simulink model "untitled"  (R2019a)
settings: Solver=VariableStepAuto  StartTime=0.0  StopTime=1  RelTol=1e-3
undefined symbols (not defined in the file or in its folder): a, myconv, tau
libraries: simulink x1, cstblocks x1
settings Model: Creator=70654  LastModifiedBy=70654
settings SolverCC: AlgebraicLoopSolver=LineSearch

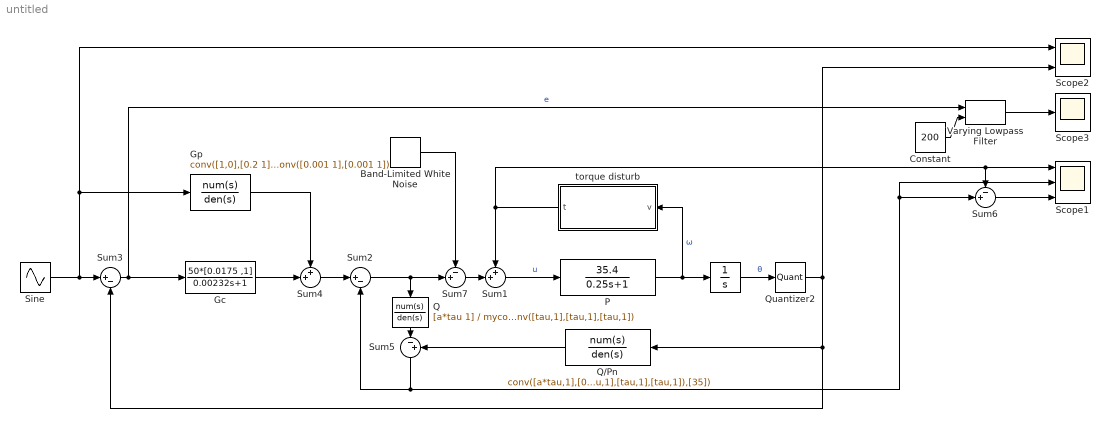
== system untitled ==
  " " : Integrator
  "                                                         P" : TransferFcn  Numerator=[35.4]  Denominator=[0.25 1]
  Band-Limited White Noise : simulink/Sources/Band-Limited White Noise  Cov=[1]  Ts=0.001  seed=[23341]
  Constant : Constant  Value=200
  Gc : TransferFcn  Numerator=50*[0.0175 ,1]  Denominator=[0.00232,1]
  Gp : TransferFcn  Numerator=conv([1,0],[0.2 1])  Denominator=35*conv([0.001 1],[0.001 1])
  Q : TransferFcn  Numerator=[a*tau 1]  Denominator=myconv([tau,1],[tau,1],[tau,1])
  Q/Pn : TransferFcn  Numerator=conv([a*tau,1],[0.2,1,0])  Denominator=conv(myconv([tau,1],[tau,1],[tau,1]),[35])
  Quantizer2 : Quantizer  QuantizationInterval=1/1800
  Scope1 : Scope  NumInputPorts=3
  Scope2 : Scope  NumInputPorts=2
  Scope3 : Scope
  "Sine " : Sin  Amplitude=0.5  Frequency=10*2*pi  SampleTime=0.001  mask(DiscretizedSource){}
      mask init:
      | %zoh
  Sum1 : Sum  Inputs=++|
  Sum2 : Sum  Inputs=|+-
  Sum3 : Sum  Inputs=|+-
  Sum4 : Sum  Inputs=++|
  Sum5 : Sum  Inputs=|-+
  Sum6 : Sum  Inputs=-+|
  Sum7 : Sum  Inputs=-+|
  Varying Lowpass Filter : cstblocks/Linear Parameter Varying/Varying Lowpass Filter  N=1
      settings: SourceProductName=Control System Toolbox
  torque disturb : MATLAB Function  TreatAsAtomicUnit=on
  wires:
  "                                                         P"/1 -> " "/1, torque disturb/1(v)  "ω"
  Sum3/1 -> Varying Lowpass Filter/1, Gc/1  "e"
  " "/1 -> Quantizer2/1  "θ"
  Quantizer2/1 -> Scope2/2, Q/Pn/1, Sum3/2
  Sum1/1 -> "                                                         P"/1  "u"
  "Sine "/1 -> Gp/1, Scope2/1, Sum3/1
  torque disturb/1(t) -> Sum1/1, Scope1/1, Sum6/1
  Gp/1 -> Sum4/1
  Q/1 -> Sum5/1
  Q/Pn/1 -> Sum5/2
  Sum5/1 -> Sum2/2, Scope1/2, Sum6/2
  Sum2/1 -> Sum7/2, Q/1
  Gc/1 -> Sum4/2
  Sum6/1 -> Scope1/3
  Band-Limited White Noise/1 -> Sum7/1
  Sum4/1 -> Sum2/1
  Sum7/1 -> Sum1/2
  Varying Lowpass Filter/1 -> Scope3/1
  Constant/1 -> Varying Lowpass Filter/2

== matlab function untitled/torque disturb ==
  data: v input; t output
function t = fcn(v)
t = 0.8*v + (1 + 9*exp(-2.2*abs(v)))*sign(v);
end
